simulink model "eccentricSingularROE"  (R2023b)
settings: Solver=ode4  StartTime=0.0  StopTime=10.0  FixedStep=dt  RelTol=1e-3
settings Model: Creator=ndelurgio  LastModifiedBy=ndelurgio

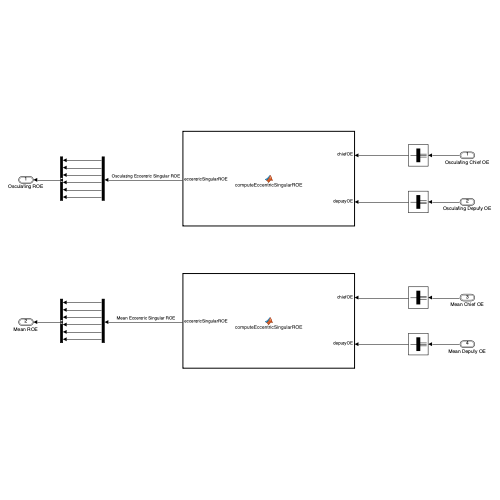
[thumbnail: Simulink's stored preview of the top-level diagram]
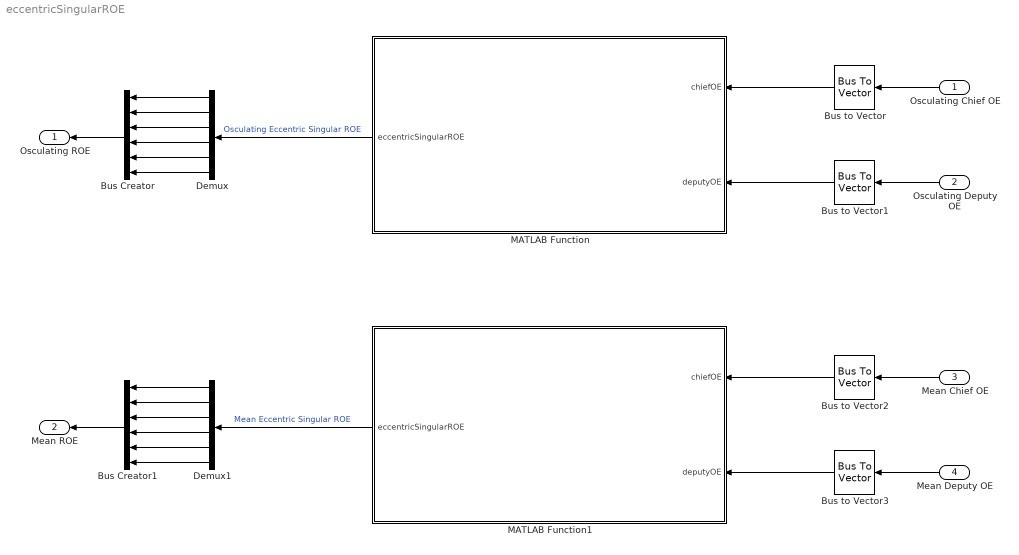
== system eccentricSingularROE ==
  Osculating Chief OE : Inport  OutDataTypeStr=Bus: osculatingOrbitElements
  Osculating Deputy OE : Inport  Port=2  OutDataTypeStr=Bus: osculatingOrbitElements
  Mean Chief OE : Inport  Port=3  OutDataTypeStr=Bus: meanOrbitElements
  Mean Deputy OE : Inport  Port=4  OutDataTypeStr=Bus: meanOrbitElements
  Bus Creator : BusCreator  Inputs=6  OutDataTypeStr=Bus: eccentricSingularROE
  Bus Creator1 : BusCreator  Inputs=6  OutDataTypeStr=Bus: eccentricSingularROE
  Bus to Vector{,1..3} (4 alike) : BusToVector
  Demux : Demux  Outputs=6
  Demux1 : Demux  Outputs=6
  MATLAB Function : MATLAB Function  TreatAsAtomicUnit=on
  MATLAB Function1 : MATLAB Function  TreatAsAtomicUnit=on
  Osculating ROE : Outport  OutDataTypeStr=Bus: eccentricSingularROE
  Mean ROE : Outport  Port=2  OutDataTypeStr=Bus: eccentricSingularROE
  wires:
  Osculating Chief OE/1 -> Bus to Vector/1
  Osculating Deputy OE/1 -> Bus to Vector1/1
  Bus to Vector/1 -> MATLAB Function/1(chiefOE)
  Bus to Vector1/1 -> MATLAB Function/2(deputyOE)
  MATLAB Function/1(eccentricSingularROE) -> Demux/1  "Osculating Eccentric Singular ROE"
  Demux/1 -> Bus Creator/1
  Demux/2 -> Bus Creator/2
  Demux/3 -> Bus Creator/3
  Demux/4 -> Bus Creator/4
  Demux/5 -> Bus Creator/5
  Demux/6 -> Bus Creator/6
  Bus Creator/1 -> Osculating ROE/1
  Mean Deputy OE/1 -> Bus to Vector3/1
  Demux1/2 -> Bus Creator1/2
  Demux1/6 -> Bus Creator1/6
  Mean Chief OE/1 -> Bus to Vector2/1
  Demux1/4 -> Bus Creator1/4
  Demux1/1 -> Bus Creator1/1
  MATLAB Function1/1(eccentricSingularROE) -> Demux1/1  "Mean Eccentric Singular ROE"
  Demux1/3 -> Bus Creator1/3
  Bus to Vector3/1 -> MATLAB Function1/2(deputyOE)
  Bus Creator1/1 -> Mean ROE/1
  Demux1/5 -> Bus Creator1/5
  Bus to Vector2/1 -> MATLAB Function1/1(chiefOE)

== matlab function eccentricSingularROE/MATLAB Function ==
  data: chiefOE input; eccentricSingularROE output; deputyOE input
function eccentricSingularROE = computeEccentricSingularROE(chiefOE, deputyOE)

eccentricSingularROE = computeEccentricSingularROE(chiefOE, deputyOE);

end

== matlab function eccentricSingularROE/MATLAB Function1 ==
  data: chiefOE input; eccentricSingularROE output; deputyOE input
function eccentricSingularROE = computeEccentricSingularROE(chiefOE, deputyOE)

eccentricSingularROE = computeEccentricSingularROE(chiefOE, deputyOE);

end
